simulink library "csc_thl_thrusters_mtv_lib"  (R2014b)
settings: Solver=ode45  StartTime=0.0  StopTime=10.0  RelTol=1e-3
undefined symbols (not defined in the file or in its folder): mpl_gn2_mass_initial
libraries: simulink x1, util_info_lib x1, csc_tdl_thruster_dynamics_collection_mtv_lib x1, csu_tfl_thruster_forces_mtv_lib x1, csu_tpl_thruster_propellant_mtv_lib x1
settings Model: Creator=Nilesh  LastModifiedBy=mstewart

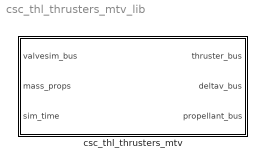
== system csc_thl_thrusters_mtv_lib ==
  csc_thl_thrusters_mtv : Subsystem

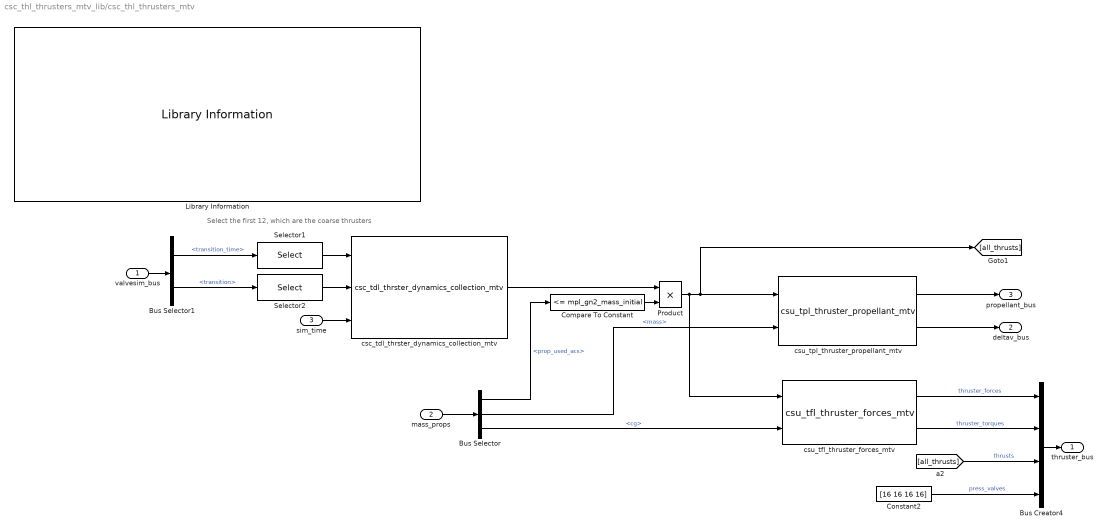
== system csc_thl_thrusters_mtv_lib/csc_thl_thrusters_mtv ==
  note: Select the first 12, which are the coarse thrusters
  valvesim_bus : Inport
  mass_props : Inport  Port=2
  sim_time : Inport  Port=3
  Bus Creator4 : BusCreator  OutDataTypeStr=Bus: actuator_mtv_msg_t
  Bus Selector : BusSelector  OutputSignals=prop_used_acs,mass,cg
  Bus Selector1 : BusSelector  OutputSignals=transition_time,transition
  Compare To Constant : simulink/Logic and Bit Operations/Compare To Constant  relop=<=  const=mpl_gn2_mass_initial  OutDataTypeStr=uint8
  Constant2 : Constant  Value=[16 16 16 16]  OutDataTypeStr=uint8
  Library Information : util_info_lib/Library Information  owner='NONE'
  Product : Product
  Selector1 : Selector  InputPortWidth=22  Indices=[1:12]
  Selector2 : Selector  InputPortWidth=22  Indices=[1:12]
  csc_tdl_thrster_dynamics_collection_mtv : csc_tdl_thruster_dynamics_collection_mtv_lib/csc_tdl_thrster_dynamics_collection_mtv  SystemSampleTime=-1
  csu_tfl_thruster_forces_mtv : csu_tfl_thruster_forces_mtv_lib/csu_tfl_thruster_forces_mtv
  csu_tpl_thruster_propellant_mtv : csu_tpl_thruster_propellant_mtv_lib/csu_tpl_thruster_propellant_mtv
  thruster_bus : Outport
  deltav_bus : Outport  Port=2
  propellant_bus : Outport  Port=3
  wires:
  Constant2/1 -> Bus Creator4/4  "press_valves"
  Bus Selector/1 -> Compare To Constant/1  "<prop_used_acs>"
  Selector2/1 -> csc_tdl_thrster_dynamics_collection_mtv/2
  Selector1/1 -> csc_tdl_thrster_dynamics_collection_mtv/1
  Compare To Constant/1 -> Product/2
  csc_tdl_thrster_dynamics_collection_mtv/1 -> Product/1
  [all_thrusts] -> Bus Creator4/3  "thrusts"
  csu_tfl_thruster_forces_mtv/1 -> Bus Creator4/1  "thruster_forces"
  csu_tfl_thruster_forces_mtv/2 -> Bus Creator4/2  "thruster_torques"
  Bus Creator4/1 -> thruster_bus/1
  Bus Selector1/1 -> Selector1/1  "<transition_time>"
  Bus Selector1/2 -> Selector2/1  "<transition>"
  csu_tpl_thruster_propellant_mtv/1 -> propellant_bus/1
  csu_tpl_thruster_propellant_mtv/2 -> deltav_bus/1
  valvesim_bus/1 -> Bus Selector1/1
  sim_time/1 -> csc_tdl_thrster_dynamics_collection_mtv/3
  Bus Selector/3 -> csu_tfl_thruster_forces_mtv/2  "<cg>"
  Bus Selector/2 -> csu_tpl_thruster_propellant_mtv/2  "<mass>"
  mass_props/1 -> Bus Selector/1
  Product/1 -> csu_tpl_thruster_propellant_mtv/1, [all_thrusts], csu_tfl_thruster_forces_mtv/1
